simulink model "Inseguitore_maggiore_di_zero"  (R2024b)
settings: Solver=VariableStepAuto  StartTime=0.0  StopTime=10  RelTol=1e-3
settings Model: Creator=miche  LastModifiedBy=miche

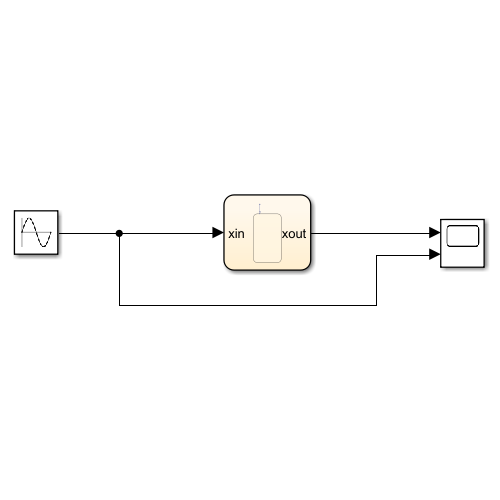
[thumbnail: Simulink's stored preview of the top-level diagram]
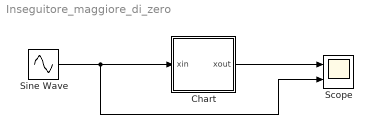
== system Inseguitore_maggiore_di_zero ==
  Chart : Stateflow chart  TreatAsAtomicUnit=on
  Scope : Scope  NumInputPorts=2
  Sine Wave : Sin  SampleTime=0
  wires:
  Sine Wave/1 -> Scope/2, Chart/1(xin)
  Chart/1(xout) -> Scope/1

== stateflow chart Inseguitore_maggiore_di_zero/Chart ==
  state Chekif
    during:
    if (xin < 0)
    xout = 0;
    else
    xout = xin;
    end
  (default) -> Chekif
  data: xin input; xout output double =0
